simulink subsystem "subsystem_gmsFriction"  (R2022a)
settings: Solver=VariableStepAuto  StartTime=0.0  StopTime=10.0  RelTol=1e-3
settings Model: Creator=Philipp  LastModifiedBy=Philipp
settings DebuggingCC: UnconnectedInputMsg=warning  UnconnectedOutputMsg=warning  UnconnectedLineMsg=warning
settings RTWCC: DLArmComputeVersion=19.05

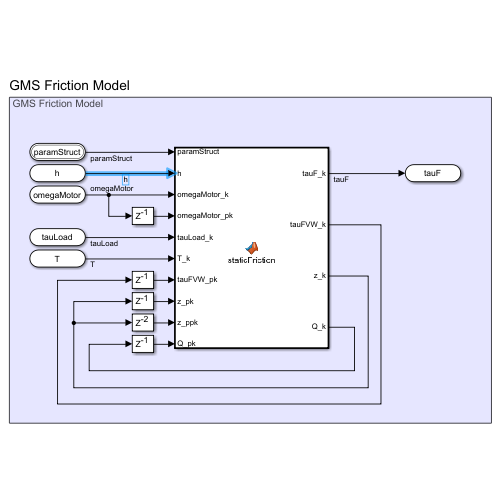
[thumbnail: Simulink's stored preview of the top-level diagram]
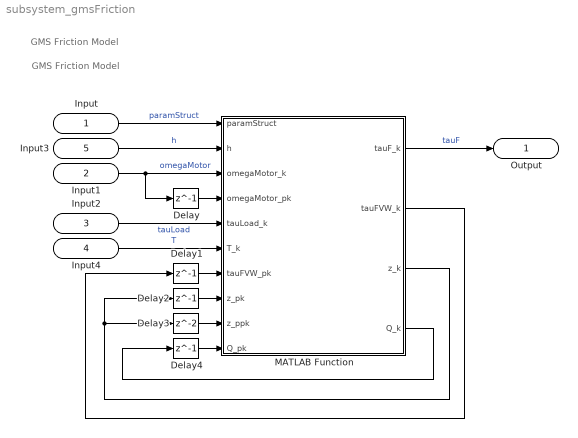
== system subsystem_gmsFriction ==
  note: GMS Friction Model
  note: GMS Friction Model
  Input : Inport  OutDataTypeStr=Bus: main_bus
  Input1 : Inport  Port=2
  Input2 : Inport  Port=3  PortDimensions=3
  Input4 : Inport  Port=4
  Input3 : Inport  Port=5
  Delay{,1..2,4} (4 alike) : Delay  DelayLength=1
  Delay3 : Delay
  MATLAB Function : MATLAB Function  TreatAsAtomicUnit=on
  Output : Outport
  wires:
  Input/1 -> MATLAB Function/1(paramStruct)  "paramStruct"
  MATLAB Function/1(tauF_k) -> Output/1  "tauF"
  Input4/1 -> MATLAB Function/6(T_k)  "T"
  Input2/1 -> MATLAB Function/5(tauLoad_k)  "tauLoad"
  Input1/1 -> Delay/1, MATLAB Function/3(omegaMotor_k)  "omegaMotor"
  Delay/1 -> MATLAB Function/4(omegaMotor_pk)
  Input3/1 -> MATLAB Function/2(h)  "h"
  Delay1/1 -> MATLAB Function/7(tauFVW_pk)
  MATLAB Function/2(tauFVW_k) -> Delay1/1
  MATLAB Function/3(z_k) -> Delay2/1, Delay3/1
  Delay3/1 -> MATLAB Function/9(z_ppk)
  Delay2/1 -> MATLAB Function/8(z_pk)
  Delay4/1 -> MATLAB Function/10(Q_pk)
  MATLAB Function/4(Q_k) -> Delay4/1

== matlab function subsystem_gmsFriction/MATLAB Function ==
  data: paramStruct input; h input; omegaMotor_k input; omegaMotor_pk input; tauLoad_k input; T_k input; tauFVW_pk input; tauF_k output; z_pk input; z_ppk input; tauFVW_k output; z_k output; Q_pk input; Q_k output
function [tauF_k, tauFVW_k, z_k, Q_k] = staticFriction(paramStruct, h, omegaMotor_k, omegaMotor_pk, tauLoad_k, T_k, tauFVW_pk, z_pk, z_ppk, Q_pk)

i_g = paramStruct.robot.i_g;

% Convert to deg
omegaMotorDeg_k = omegaMotor_k .* (180/pi);
omegaMotorDeg_pk = omegaMotor_pk .* (180/pi);

[tauF_k, tauFVW_k, z_k, Q_k] = ...
    gmsFriction_model_midpoint(paramStruct, h, omegaMotorDeg_k, omegaMotorDeg_pk, tauFVW_pk, tauLoad_k, T_k, z_pk, z_ppk, Q_pk);
tauF_k = tauF_k .* i_g;
